simulink model "ModelGenericDrive"  (R2020b)
settings: Solver=FixedStepAuto  StartTime=0.0  StopTime=Inf  FixedStep=0.010  RelTol=1e-3
settings Model: Creator=kaebi  LastModifiedBy=kaebi
settings OptimizationCC: DefaultParameterBehavior=Inlined  LocalBlockOutputs=off
settings RTWCC: Description=TwinCAT GRT Target  SystemTargetFile=TwinCatGrt.tlc  TemplateMakefile=tcgrt_msbuild.tmf  TargetLang=C++
settings STFCustomTargetCC: TargetLangStandard=C++03 (ISO)  ConcurrentExecutionCompliant=off  CombineOutputUpdateFcns=on  CodeInterfacePackaging=Reusable function  GRTInterface=off  GenerateAllocFcn=on  SystemTargetFile=TwinCatGrt.tlc
settings GRTTargetCC: TargetLangStandard=C++03 (ISO)  ParMdlRefBuildCompliant=off  CompOptLevelCompliant=off  ConcurrentExecutionCompliant=off  MatFileLogging=off  CodeInterfacePackaging=Reusable function  GenerateAllocFcn=on  UseToolchainInfoCompliant=off  ExtModeMexFile=TcExtModeClient
settings ConfigComp: PLC_TargetIDE=codesys23

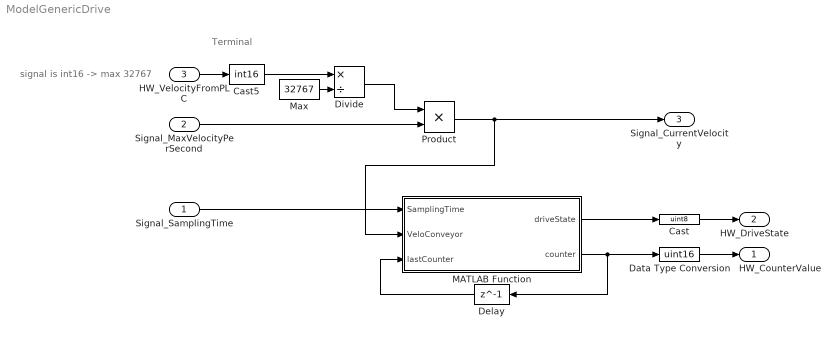
== system ModelGenericDrive ==
  note: Terminal
  note: signal is int16 -> max 32767
  Signal_SamplingTime : Inport
  Signal_MaxVelocityPerSecond : Inport  Port=2
  HW_VelocityFromPLC : Inport  Port=3
  Cast : DataTypeConversion  OutDataTypeStr=uint8
  Cast5 : DataTypeConversion  OutDataTypeStr=int16
  Data Type Conversion : DataTypeConversion  OutDataTypeStr=uint16  SaturateOnIntegerOverflow=on
  Delay : Delay  DelayLength=1
  Divide : Product  Inputs=*/
  MATLAB Function : MATLAB Function  TreatAsAtomicUnit=on
  Max : Constant  Value=32767
  Product : Product
  HW_CounterValue : Outport
  HW_DriveState : Outport  Port=2
  Signal_CurrentVelocity : Outport  Port=3
  wires:
  Signal_SamplingTime/1 -> MATLAB Function/1(SamplingTime)
  Delay/1 -> MATLAB Function/3(lastCounter)
  MATLAB Function/2(counter) -> Delay/1, Data Type Conversion/1
  Product/1 -> Signal_CurrentVelocity/1, MATLAB Function/2(VeloConveyor)
  HW_VelocityFromPLC/1 -> Cast5/1
  Divide/1 -> Product/1
  Signal_MaxVelocityPerSecond/1 -> Product/2
  Max/1 -> Divide/2
  Cast5/1 -> Divide/1
  Cast/1 -> HW_DriveState/1
  MATLAB Function/1(driveState) -> Cast/1
  Data Type Conversion/1 -> HW_CounterValue/1

== matlab function ModelGenericDrive/MATLAB Function ==
  data: driveState output; SamplingTime input; VeloConveyor input; counter output; lastCounter input
function [driveState,counter] = fcn(SamplingTime, VeloConveyor, lastCounter)
%%
%    VeloConveyor in Unit/s
%    SamplingTime in s
%    lastCounter 1count = 0.0001 Unit

%%
driveState = uint8(0);
driveState = bitset(driveState,1,1);    % Ready to enable
driveState = bitset(driveState,2,1);    % Ready 
if (VeloConveyor > 0)
    driveState = bitset(driveState,5,1);    % Moving Positive
elseif (VeloConveyor < 0)
    driveState = bitset(driveState,6,1);    % Moving Negative
end

diff = VeloConveyor*SamplingTime*10000;
if (lastCounter+diff >= 65535)
    counter = lastCounter+diff -65535;
else
    counter = lastCounter + VeloConveyor*SamplingTime*10000;
end

end
